simulink model "suspension_test"  (R2020b)
settings: Solver=VariableStepAuto  StartTime=0.0  StopTime=10.0  RelTol=1e-3
values from neighbouring files (symbols this model uses):
  b = 1    [accel_jerk_ctrl_testbed.m]    (also in halfcarparameters.mat = 1.5)
  k = 1    [accel_jerk_ctrl_testbed.m]
  m = 1    [accel_jerk_ctrl_testbed.m]
settings Model: Creator=sharad  LastModifiedBy=anishabhangui
settings DataIOCC: ReturnWorkspaceOutputs=off
settings DebuggingCC: ArithmeticOperatorsInVariantConditions=warning
settings SFSimCC: SimUseLocalCustomCode=off  CustomCodeUndefinedFunction=UseInterfaceOnly
settings RTWCC: RTWUseLocalCustomCode=off

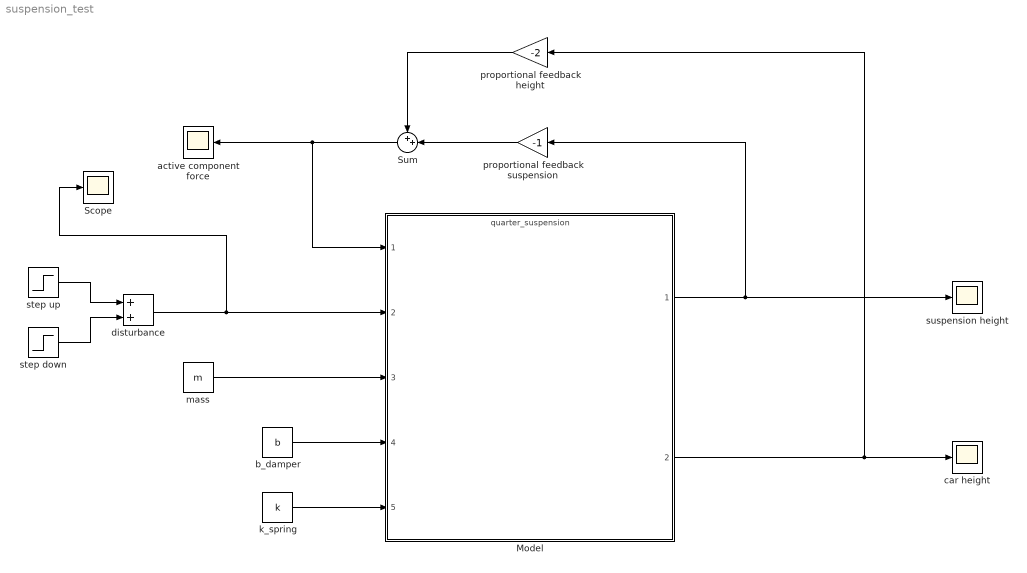
== system suspension_test ==
  Model : ModelReference  ModelNameDialog=quarter_suspension.slx  SimulationMode=Normal  ModelReferenceVersion=6.1
  Scope : Scope
  Sum : Sum  Inputs=++|
  active component force : Scope
  b_damper : Constant  Value=b
  car height : Scope
  disturbance : Sum
  "k_spring " : Constant  Value=k
  mass : Constant  Value=m
  proportional feedback height : Gain  Gain=-2
  proportional feedback suspension : Gain  Gain=-1
  step down : Step  After=-1  SampleTime=0
  step up : Step  Time=0  SampleTime=0
  suspension height : Scope
  wires:
  "k_spring "/1 -> Model/5
  mass/1 -> Model/3
  step up/1 -> disturbance/1
  step down/1 -> disturbance/2
  disturbance/1 -> Scope/1, Model/2
  Model/1 -> suspension height/1, proportional feedback suspension/1
  Model/2 -> proportional feedback height/1, car height/1
  b_damper/1 -> Model/4
  Sum/1 -> Model/1, active component force/1
  proportional feedback height/1 -> Sum/1
  proportional feedback suspension/1 -> Sum/2
